simulink model "con_ESTNavigation"  (R2017a)
settings: Solver=FixedStepAuto  StartTime=0.0  StopTime=24  FixedStep=0.1  RelTol=1e-3
settings Model: Creator=xiaodong  LastModifiedBy=xiaodong
settings DataIOCC: SaveFormat=Array  SaveOutput=off  SignalLogging=off  DSMLogging=off  SaveTime=off

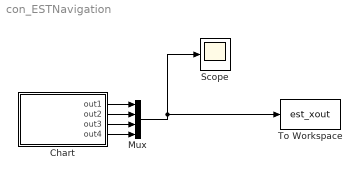
== system con_ESTNavigation ==
  Chart : Stateflow chart  TreatAsAtomicUnit=on
  Mux : Mux
  Scope : Scope
  To Workspace : ToWorkspace  VariableName=est_xout  SampleTime=-1
  wires:
  Mux/1 -> Scope/1, To Workspace/1
  Chart/1(out1) -> Mux/1
  Chart/2(out2) -> Mux/2
  Chart/3(out3) -> Mux/3
  Chart/4(out4) -> Mux/4

== stateflow chart con_ESTNavigation/Chart ==
  settings: updateMethod=CONTINUOUS
  state M2
    entry:
    A1 = [0,  0,  0.1,  0;
    0,  0,  0,  0.1;
    0,  0,  -0.12  0.01;
    0,  0,  0.01  -0.12];
    B1 =[0; 0; 0.01; -0.12];
    during:
    x1_dot = A1(1,1)*x1+A1(1,2)*x2+A1(1,3)*x3+A1(1,4)*x4+B1(1);
    x2_dot = A1(2,1)*x1+A1(2,2)*x2+A1(2,3)*x3+A1(2,4)*x4+B1(2);
    x3_dot = A1(3,1)*x1+A1(3,2)*x2+A1(3,3)*x3+A1(3,4)*x4+B1(3);
    x4_dot = A1(4,1)*x1+A1(4,2)*x2+A1(4,3)*x3+A1(4,4)*x4+B1(4);
    out1 = x1;
    out2 = x2;
    out3 = x3;
    out4 = x4;
  state M3
    entry:
    A3 =[0,  0,  0.1,  0;
    0,  0,  0,  0.1;
    0,  0,  -0.12  0.01;
    0,  0,  0.01  -0.12];
    B3 =[0.0000; 0.0000; 0.0919; -0.0919];
    during:
    x1_dot = A3(1,1)*x1+A3(1,2)*x2+A3(1,3)*x3+A3(1,4)*x4+B3(1);
    x2_dot = A3(2,1)*x1+A3(2,2)*x2+A3(2,3)*x3+A3(2,4)*x4+B3(2);
    x3_dot = A3(3,1)*x1+A3(3,2)*x2+A3(3,3)*x3+A3(3,4)*x4+B3(3);
    x4_dot = A3(4,1)*x1+A3(4,2)*x2+A3(4,3)*x3+A3(4,4)*x4+B3(4);
    out1 = x1;
    out2 = x2;
    out3 = x3;
    out4 = x4;
  state M41
    entry:
    entry:
    A2 = [0,  0,  0.1,  0;
    0,  0,  0,  0.1;
    0,  0,  -0.12  0.01;
    0,  0,  0.01  -0.12];
    B2 =[0; 0; 0.12; -0.01];
    during:
    x1_dot = A2(1,1)*x1+A2(1,2)*x2+A2(1,3)*x3+A2(1,4)*x4+B2(1);
    x2_dot = A2(2,1)*x1+A2(2,2)*x2+A2(2,3)*x3+A2(2,4)*x4+B2(2);
    x3_dot = A2(3,1)*x1+A2(3,2)*x2+A2(3,3)*x3+A2(3,4)*x4+B2(3);
    x4_dot = A2(4,1)*x1+A2(4,2)*x2+A2(4,3)*x3+A2(4,4)*x4+B2(4);
    out1 = x1;
    out2 = x2;
    out3 = x3;
    out4 = x4;
  state M42
    entry:
    A1 = [0,  0,  0.1,  0;
    0,  0,  0,  0.1;
    0,  0,  -0.12  0.01;
    0,  0,  0.01  -0.12];
    B1 =[0; 0; 0.01; -0.12];
    during:
    x1_dot = A1(1,1)*x1+A1(1,2)*x2+A1(1,3)*x3+A1(1,4)*x4+B1(1);
    x2_dot = A1(2,1)*x1+A1(2,2)*x2+A1(2,3)*x3+A1(2,4)*x4+B1(2);
    x3_dot = A1(3,1)*x1+A1(3,2)*x2+A1(3,3)*x3+A1(3,4)*x4+B1(3);
    x4_dot = A1(4,1)*x1+A1(4,2)*x2+A1(4,3)*x3+A1(4,4)*x4+B1(4);
    out1 = x1;
    out2 = x2;
    out3 = x3;
    out4 = x4;
  state M43
    during:
    out1 = -1;
    out2 = -1;
    out3 = -1;
    out4 = -1;
  state M1
    entry:
    A2 = [0,  0,  0.1,  0;
    0,  0,  0,  0.1;
    0,  0,  -0.12  0.01;
    0,  0,  0.01  -0.12];
    B2 =[0; 0; 0.12; -0.01];
    during:
    x1_dot = A2(1,1)*x1+A2(1,2)*x2+A2(1,3)*x3+A2(1,4)*x4+B2(1);
    x2_dot = A2(2,1)*x1+A2(2,2)*x2+A2(2,3)*x3+A2(2,4)*x4+B2(2);
    x3_dot = A2(3,1)*x1+A2(3,2)*x2+A2(3,3)*x3+A2(3,4)*x4+B2(3);
    x4_dot = A2(4,1)*x1+A2(4,2)*x2+A2(4,3)*x3+A2(4,4)*x4+B2(4);
    out1 = x1;
    out2 = x2;
    out3 = x3;
    out4 = x4;
  state M44
    during:
    out1 = -1;
    out2 = -1;
    out3 = -1;
    out4 = -1;
  M3 -> M1 [order 3] : [0.0083*x1-1.0007*x2-0.0166*x3+ 0.0139*x4+ 1>=0]
  (default) -> M1 : {x1 = 0.4; x2= 0.62; x3= 0.5; x4= 1;}
  M1 -> M2 [order 1] : [ 0.0049*x1-0.9980*x2-0.0134*x3+ 0.0217*x4+ 1<=0]
  M3 -> M41 [order 1] : [-0.0045*x1-0.4971*x2+ 0.0011*x3+ 0.0064*x4+ 1<=0]
  M2 -> M3 [order 2] : [-1.0065*x1+ 0.0031*x2+ 0.0201*x3-0.0028*x4+ 1<=0]
  M41 -> M42 : [-0.4904*x1-0.0049*x2+ 0.0030*x3+ 1<=0]
  M42 -> M43 : [0.0054*x1-0.9710*x2-0.0176*x3+ 0.0521*x4+ 1>=0]
  M2 -> M1 [order 1] : [ 0.0011*x1-1.0070*x2+ 0.0159*x3+ 0.0126*x4+1>=0]
  M3 -> M42 [order 2] : [-0.4784*x1+ 0.0019*x2-0.0449*x3+ 0.0168*x4+ 1<=0]
  M1 -> M44 [order 2] : [-0.5018*x1+ 0.0067*x3-0.0030*x4+ 1<=0]
  data: A2 local size=[4,4]; A1 local size=[4,4]; A3 local size=[4,4]; out1 output; out2 output; out3 output; out4 output; B1 local size=[4,1]; B2 local size=[4,1]; B3 local size=[4,1]; x1 local; x2 local; x3 local; x4 local
  data x1 settings: updateMethod=SF_CONTINUOUS_TIME_DATA
  data x2 settings: updateMethod=SF_CONTINUOUS_TIME_DATA
  data x3 settings: updateMethod=SF_CONTINUOUS_TIME_DATA
  data x4 settings: updateMethod=SF_CONTINUOUS_TIME_DATA
